simulink model "NeuromorphicDogGait_WalksBackwards"  (R2022b)
settings: Solver=ode4  StartTime=0.0  StopTime=10  FixedStep=1e-3  RelTol=1e-3
undefined symbols (not defined in the file): t1, t2, Vus0
libraries: vexv5lib x24, vexcommonlib x16, Vex_V5_Simulink_Expansion x8
(part 1 of 3)
settings Model: Creator=Serious Chimp  LastModifiedBy=Serious Chimp
settings DataIOCC: SaveFormat=StructureWithTime  InspectSignalLogs=on
settings OptimizationCC: EnhancedBackFolding=on  PassReuseOutputArgsAs=Individual arguments  ZeroExternalMemoryAtStartup=off  ZeroInternalMemoryAtStartup=off  MaxStackSize=64  OptimizeBlockOrder=speed  DifferentSizesBufferReuse=on  OptimizationCustomize=off  EfficientTunableParamExpr=on
settings DebuggingCC: ParameterTunabilityLossMsg=error
settings HardwareCC: ProdBitPerPointer=32  ProdBitPerSizeT=32  ProdBitPerPtrDiffT=32  ProdLargestAtomicInteger=Long  ProdLargestAtomicFloat=Double  ProdWordSize=32  ProdHWDeviceType=ARM Compatible->ARM Cortex  UseEmbeddedCoderFeatures=off
settings SFSimCC: MATLABDynamicMemAlloc=off
settings RTWCC: Description=Embedded Coder  SystemTargetFile=ert.tlc  HardwareBoard=VEX V5 Robot Brain  TLCOptions="-aInlineSetEventsForThisBaseRateFcn=TLC_FALSE -aSuppressMultiTaskScheduler=TLC_FALSE  -aRateBasedStepFcn=0"  TemplateMakefile=ert_default_tmf  Toolchain=GNU Tools for ARM Embedded Processors
settings CodeAppCC: ForceParamTrailComments=on  IgnoreCustomStorageClasses=off  OperatorAnnotations=on  SimulinkDataObjDesc=on  SFDataObjDesc=on  InsertBlockDesc=on
settings ERTTargetCC: SupportNonInlinedSFcns=on  ExtModeTransport=3  ExtModeStaticAlloc=on  ExtModeStaticAllocSize=2048  ExtModeMexFile=ext_xcp  ExtModeIntrfLevel=Level2 - Open

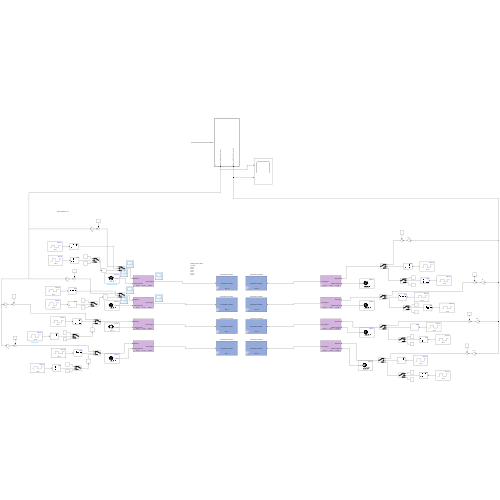
[thumbnail: Simulink's stored preview of the top-level diagram]
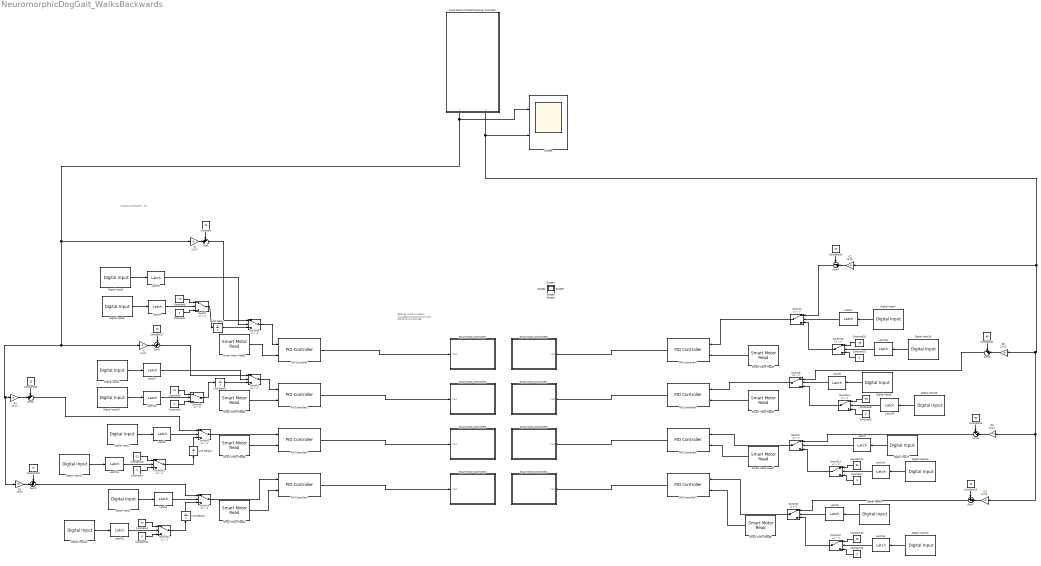
== system NeuromorphicDogGait_WalksBackwards ==
  note: Output amplitude ~ 19
  note: Settings used in videos:
      | k1=1200
      | k2=10
      | k3=10
      | C=15
      | D=23
      | t1=1.5
      | t2=190
  -C{,1..3} (4 alike) : Gain  Gain=15/19
  Constant : Constant  Value=70
  Constant{1..3,5,7,11..12,15} (8 alike) : Constant  Value=0
  Constant10 : Constant  Value=-13
  Constant13 : Constant  Value=15
  Constant14 : Constant  Value=90
  Constant16 : Constant  Value=-15
  Constant17 : Constant  Value=13
  Constant18 : Constant  Value=13
  Constant19 : Constant  Value=70
  Constant20 : Constant  Value=15
  Constant21 : Constant  Value=90
  Constant22 : Constant  Value=90
  Constant23 : Constant  Value=15
  Constant4 : Constant  Value=70
  Constant6 : Constant  Value=-90
  Constant8 : Constant  Value=-70
  Constant9 : Constant  Value=13
  D{,1..3} (4 alike) : Gain  Gain=23/19
  Digital Input{1..8} (8 alike) : vexv5lib/Sensors/Digital Input  smartPort3wire=None  port=H  SampleTime=0.2
  Digital Input{9..16} (8 alike) : vexv5lib/Sensors/Digital Input  smartPort3wire=None  port=A  SampleTime=0.2
  Latch{1..16} (16 alike) : vexcommonlib/Latch  output0=off  BlockPlatform=vexv5
      settings: LibrarySourceBlock=vexv5lib/Utilities/Latch
  PID Controller : Vex_V5_Simulink_Expansion/Core Blocks/PID Controller  KP=k1  KI=k3  KD=k2  LimitOutput=off  limitHigh=10  limitLow=10  AntiWindupMode=none  kb=0
      settings: SourceProductName=Vex V5 Simulink Expansion
  PID Controller{1..7} (7 alike) : Vex_V5_Simulink_Expansion/Core Blocks/PID Controller  KP=k1  KI=k3  KD=k2  LimitOutput=off  limitHigh=0  limitLow=0  AntiWindupMode=none  kb=0
      settings: SourceProductName=Vex V5 Simulink Expansion
  Quad-Centre (Closed Coupling) Oscillator : Subsystem  TreatAsAtomicUnit=on  mask{tau_s_A=t1, tau_us_A=t2, GB_A=-40, tau_s_B=t1, tau_us_B=t2, GB_B=-20, tau_s_C=t1, tau_us_C=t2, GB_C=-20, tau_s_D=t1, tau_us_D=t2, GB_D=-40, pain_threshold=2, pain_intensity=2, delay=0}
      mask prompts: tau_s_A "A - tau_s"; tau_us_A "A - tau_us"; GB_A "A - Inhibitory Synapse Threshold, GB_A"; tau_s_B "B - tau_s"; tau_us_B "B - tau_us"; GB_B "B - Inhibitory Synapse Threshold, GB_B"; tau_s_C "C - tau_s"; tau_us_C "C - tau_us"; GB_C "C - Inhibitory Synapse Threshold, GB_C"; tau_s_D "D - tau_s"; tau_us_D "D - tau_us"; GB_D "D - Inhibitory Synapse Threshold, GB_D"; pain_threshold "Range of Motion Pain Threshold, pain_threshold"; pain_intensity "Rang of Motion Intensity, pain_intensity"
  Scope6 : Scope  NumInputPorts=2
  Smart Motor Controller1 : Subsystem  AncestorBlock=Vex_V5_Simulink_Expansion/Core Blocks/Smart Motor Controller  mask(Smart Motor Controller){motorPort=19, OperationMode=Advanced Control, MotorBrakeMode=Coast}
      mask prompts: motorPort "Smart Port:"; OperationMode "Control Mode:"; MotorBrakeMode "Braking Mode:"
      mask help: Controls the Vex Smart Motor via the chosen method.
      mask TypeOptions motorPort: Advanced_SmartMotorWrite/motorPort
      mask TypeOptions OperationMode: Advanced_SmartMotorWrite/OperationMode
      mask TypeOptions MotorBrakeMode: Advanced_SmartMotorWrite/MotorBrakeMode
      mask DialogControl Container3 Prompt: Smart Motor Configuration
      mask Display:
      | %mode = get_param(gcb, 'control');
      | port = get_param(gcb, 'motorPort');
      | %text(0.3,0.45,[mode]);
      | 
      | text(0.5,0.5, 'Smart Motor Controller','HorizontalAlignment','center');
      | text(0.42,0.15, ['Port: ',port]);
  Smart Motor Controller2 : Subsystem  AncestorBlock=Vex_V5_Simulink_Expansion/Core Blocks/Smart Motor Controller  mask(Smart Motor Controller){motorPort=9, OperationMode=Advanced Control, MotorBrakeMode=Coast}
      mask prompts: motorPort "Smart Port:"; OperationMode "Control Mode:"; MotorBrakeMode "Braking Mode:"
      mask help: Controls the Vex Smart Motor via the chosen method.
      mask TypeOptions motorPort: Advanced_SmartMotorWrite/motorPort
      mask TypeOptions OperationMode: Advanced_SmartMotorWrite/OperationMode
      mask TypeOptions MotorBrakeMode: Advanced_SmartMotorWrite/MotorBrakeMode
      mask DialogControl Container3 Prompt: Smart Motor Configuration
      mask Display:
      | %mode = get_param(gcb, 'control');
      | port = get_param(gcb, 'motorPort');
      | %text(0.3,0.45,[mode]);
      | 
      | text(0.5,0.5, 'Smart Motor Controller','HorizontalAlignment','center');
      | text(0.42,0.15, ['Port: ',port]);
  Smart Motor Controller3 : Subsystem  AncestorBlock=Vex_V5_Simulink_Expansion/Core Blocks/Smart Motor Controller  mask(Smart Motor Controller){motorPort=1, OperationMode=Advanced Control, MotorBrakeMode=Coast}
      mask prompts: motorPort "Smart Port:"; OperationMode "Control Mode:"; MotorBrakeMode "Braking Mode:"
      mask help: Controls the Vex Smart Motor via the chosen method.
      mask TypeOptions motorPort: Advanced_SmartMotorWrite/motorPort
      mask TypeOptions OperationMode: Advanced_SmartMotorWrite/OperationMode
      mask TypeOptions MotorBrakeMode: Advanced_SmartMotorWrite/MotorBrakeMode
      mask DialogControl Container3 Prompt: Smart Motor Configuration
      mask Display:
      | %mode = get_param(gcb, 'control');
      | port = get_param(gcb, 'motorPort');
      | %text(0.3,0.45,[mode]);
      | 
      | text(0.5,0.5, 'Smart Motor Controller','HorizontalAlignment','center');
      | text(0.42,0.15, ['Port: ',port]);
  Smart Motor Controller4 : Subsystem  AncestorBlock=Vex_V5_Simulink_Expansion/Core Blocks/Smart Motor Controller  mask(Smart Motor Controller){motorPort=11, OperationMode=Advanced Control, MotorBrakeMode=Coast}
      mask prompts: motorPort "Smart Port:"; OperationMode "Control Mode:"; MotorBrakeMode "Braking Mode:"
      mask help: Controls the Vex Smart Motor via the chosen method.
      mask TypeOptions motorPort: Advanced_SmartMotorWrite/motorPort
      mask TypeOptions OperationMode: Advanced_SmartMotorWrite/OperationMode
      mask TypeOptions MotorBrakeMode: Advanced_SmartMotorWrite/MotorBrakeMode
      mask DialogControl Container3 Prompt: Smart Motor Configuration
      mask Display:
      | %mode = get_param(gcb, 'control');
      | port = get_param(gcb, 'motorPort');
      | %text(0.3,0.45,[mode]);
      | 
      | text(0.5,0.5, 'Smart Motor Controller','HorizontalAlignment','center');
      | text(0.42,0.15, ['Port: ',port]);
  Smart Motor Controller5 : Subsystem  AncestorBlock=Vex_V5_Simulink_Expansion/Core Blocks/Smart Motor Controller  mask(Smart Motor Controller){motorPort=2, OperationMode=Advanced Control, MotorBrakeMode=Coast}
      mask prompts: motorPort "Smart Port:"; OperationMode "Control Mode:"; MotorBrakeMode "Braking Mode:"
      mask help: Controls the Vex Smart Motor via the chosen method.
      mask TypeOptions motorPort: Advanced_SmartMotorWrite/motorPort
      mask TypeOptions OperationMode: Advanced_SmartMotorWrite/OperationMode
      mask TypeOptions MotorBrakeMode: Advanced_SmartMotorWrite/MotorBrakeMode
      mask DialogControl Container3 Prompt: Smart Motor Configuration
      mask Display:
      | %mode = get_param(gcb, 'control');
      | port = get_param(gcb, 'motorPort');
      | %text(0.3,0.45,[mode]);
      | 
      | text(0.5,0.5, 'Smart Motor Controller','HorizontalAlignment','center');
      | text(0.42,0.15, ['Port: ',port]);
  Smart Motor Controller6 : Subsystem  AncestorBlock=Vex_V5_Simulink_Expansion/Core Blocks/Smart Motor Controller  mask(Smart Motor Controller){motorPort=12, OperationMode=Advanced Control, MotorBrakeMode=Coast}
      mask prompts: motorPort "Smart Port:"; OperationMode "Control Mode:"; MotorBrakeMode "Braking Mode:"
      mask help: Controls the Vex Smart Motor via the chosen method.
      mask TypeOptions motorPort: Advanced_SmartMotorWrite/motorPort
      mask TypeOptions OperationMode: Advanced_SmartMotorWrite/OperationMode
      mask TypeOptions MotorBrakeMode: Advanced_SmartMotorWrite/MotorBrakeMode
      mask DialogControl Container3 Prompt: Smart Motor Configuration
      mask Display:
      | %mode = get_param(gcb, 'control');
      | port = get_param(gcb, 'motorPort');
      | %text(0.3,0.45,[mode]);
      | 
      | text(0.5,0.5, 'Smart Motor Controller','HorizontalAlignment','center');
      | text(0.42,0.15, ['Port: ',port]);
  Smart Motor Controller7 : Subsystem  AncestorBlock=Vex_V5_Simulink_Expansion/Core Blocks/Smart Motor Controller  mask(Smart Motor Controller){motorPort=10, OperationMode=Advanced Control, MotorBrakeMode=Coast}
      mask prompts: motorPort "Smart Port:"; OperationMode "Control Mode:"; MotorBrakeMode "Braking Mode:"
      mask help: Controls the Vex Smart Motor via the chosen method.
      mask TypeOptions motorPort: Advanced_SmartMotorWrite/motorPort
      mask TypeOptions OperationMode: Advanced_SmartMotorWrite/OperationMode
      mask TypeOptions MotorBrakeMode: Advanced_SmartMotorWrite/MotorBrakeMode
      mask DialogControl Container3 Prompt: Smart Motor Configuration
      mask Display:
      | %mode = get_param(gcb, 'control');
      | port = get_param(gcb, 'motorPort');
      | %text(0.3,0.45,[mode]);
      | 
      | text(0.5,0.5, 'Smart Motor Controller','HorizontalAlignment','center');
      | text(0.42,0.15, ['Port: ',port]);
  Smart Motor Controller8 : Subsystem  AncestorBlock=Vex_V5_Simulink_Expansion/Core Blocks/Smart Motor Controller  mask(Smart Motor Controller){motorPort=20, OperationMode=Advanced Control, MotorBrakeMode=Coast}
      mask prompts: motorPort "Smart Port:"; OperationMode "Control Mode:"; MotorBrakeMode "Braking Mode:"
      mask help: Controls the Vex Smart Motor via the chosen method.
      mask TypeOptions motorPort: Advanced_SmartMotorWrite/motorPort
      mask TypeOptions OperationMode: Advanced_SmartMotorWrite/OperationMode
      mask TypeOptions MotorBrakeMode: Advanced_SmartMotorWrite/MotorBrakeMode
      mask DialogControl Container3 Prompt: Smart Motor Configuration
      mask Display:
      | %mode = get_param(gcb, 'control');
      | port = get_param(gcb, 'motorPort');
      | %text(0.3,0.45,[mode]);
      | 
      | text(0.5,0.5, 'Smart Motor Controller','HorizontalAlignment','center');
      | text(0.42,0.15, ['Port: ',port]);
  Smart Motor Read1 : vexv5lib/Sensors/Smart Motor Read  motorPort=10  EncoderUnit=Degrees  resetOption=No reset  additionalOutput=off  SampleTime=0.01
  Smart Motor Read2 : vexv5lib/Sensors/Smart Motor Read  motorPort=9  EncoderUnit=Degrees  resetOption=No reset  additionalOutput=off  SampleTime=0.01
  Smart Motor Read3 : vexv5lib/Sensors/Smart Motor Read  motorPort=2  EncoderUnit=Degrees  resetOption=No reset  additionalOutput=off  SampleTime=0.01
  Smart Motor Read4 : vexv5lib/Sensors/Smart Motor Read  motorPort=1  EncoderUnit=Degrees  resetOption=No reset  additionalOutput=off  SampleTime=0.01
  Smart Motor Read5 : vexv5lib/Sensors/Smart Motor Read  motorPort=20  EncoderUnit=Degrees  resetOption=No reset  additionalOutput=off  SampleTime=0.01
  Smart Motor Read6 : vexv5lib/Sensors/Smart Motor Read  motorPort=19  EncoderUnit=Degrees  resetOption=No reset  additionalOutput=off  SampleTime=0.01
  Smart Motor Read7 : vexv5lib/Sensors/Smart Motor Read  motorPort=12  EncoderUnit=Degrees  resetOption=No reset  additionalOutput=off  SampleTime=0.01
  Smart Motor Read8 : vexv5lib/Sensors/Smart Motor Read  motorPort=11  EncoderUnit=Degrees  resetOption=No reset  additionalOutput=off  SampleTime=0.01
  Sum{,2,4..5} (4 alike) : Sum  Inputs=-+|
  Sum{1,3,6..7} (4 alike) : Sum  Inputs=++|
  Switch{,1..15} (16 alike) : Switch  Criteria=u2 > Threshold  SaturateOnIntegerOverflow=off  InputSameDT=off
  Unit Delay{,1..3} (4 alike) : UnitDelay  SampleTime=-1  HasFrameUpgradeWarning=on
  Scope{,1..5} (6 alike) : Scope
  wires:
  Smart Motor Read1/1 -> PID Controller/2
  Smart Motor Read2/1 -> PID Controller1/2
  Smart Motor Read4/1 -> PID Controller3/2
  Smart Motor Read3/1 -> PID Controller2/2
  Smart Motor Read5/1 -> PID Controller4/2
  Smart Motor Read6/1 -> PID Controller5/2
  Smart Motor Read7/1 -> PID Controller6/2
  Smart Motor Read8/1 -> PID Controller7/2
  Digital Input5/1 -> Latch5/1
  Latch5/1 -> Switch5/2
  Switch5/1 -> PID Controller/1
  Switch9/1 -> Unit Delay1/1
  Digital Input1/1 -> Latch1/1
  Latch1/1 -> Switch1/2
  Switch1/1 -> PID Controller1/1
  Digital Input2/1 -> Latch2/1
  Latch2/1 -> Switch2/2
  Switch2/1 -> PID Controller2/1
  Digital Input3/1 -> Latch3/1
  Latch3/1 -> Switch3/2
  Switch3/1 -> PID Controller3/1
  Digital Input4/1 -> Latch4/1
  Latch4/1 -> Switch4/2
  Switch4/1 -> PID Controller4/1
  Digital Input6/1 -> Latch6/1
  Latch6/1 -> Switch6/2
  Switch6/1 -> PID Controller5/1
  Digital Input7/1 -> Latch7/1
  Latch7/1 -> Switch7/2
  Switch7/1 -> PID Controller6/1
  Digital Input8/1 -> Latch8/1
  Latch8/1 -> Switch8/2
  Switch8/1 -> PID Controller7/1
  Constant1/1 -> Switch/3
  Constant8/1 -> Switch/1
  Digital Input9/1 -> Latch9/1
  Latch9/1 -> Switch/2
  Constant9/1 -> Switch9/1
  Latch10/1 -> Switch9/2
  Constant2/1 -> Switch9/3
  Digital Input10/1 -> Latch10/1
  Constant10/1 -> Switch10/1
  Latch11/1 -> Switch10/2
  Constant3/1 -> Switch10/3
  Digital Input11/1 -> Latch11/1
  Constant11/1 -> Switch11/3
  Constant4/1 -> Switch11/1
  Digital Input12/1 -> Latch12/1
  Latch12/1 -> Switch11/2
  Digital Input13/1 -> Latch13/1
  Constant13/1 -> Switch12/1
  Constant12/1 -> Switch12/3
  Latch13/1 -> Switch12/2
  Digital Input14/1 -> Latch14/1
  Constant14/1 -> Switch13/1
  Constant7/1 -> Switch13/3
  Latch14/1 -> Switch13/2
  Digital Input15/1 -> Latch15/1
  Constant6/1 -> Switch14/1
  Constant5/1 -> Switch14/3
  Latch15/1 -> Switch14/2
  Digital Input16/1 -> Latch16/1
  Constant16/1 -> Switch15/1
  Constant15/1 -> Switch15/3
  Latch16/1 -> Switch15/2
  Switch/1 -> Unit Delay/1
  Switch10/1 -> Unit Delay2/1
  Unit Delay2/1 -> Switch2/3
  Unit Delay1/1 -> Switch1/3
  Unit Delay/1 -> Switch5/3
  Switch13/1 -> Switch7/3
  Switch14/1 -> Switch6/3
  Unit Delay3/1 -> Switch3/3
  Switch11/1 -> Unit Delay3/1
  Switch15/1 -> Switch4/3
  Switch12/1 -> Switch8/3
  PID Controller/1 -> Smart Motor Controller7/1(" Input")
  PID Controller1/1 -> Smart Motor Controller2/1(" Input")
  PID Controller2/1 -> Smart Motor Controller5/1(" Input")
  PID Controller3/1 -> Smart Motor Controller3/1(" Input")
  PID Controller4/1 -> Smart Motor Controller8/1(" Input")
  PID Controller5/1 -> Smart Motor Controller1/1(" Input")
  PID Controller6/1 -> Smart Motor Controller6/1(" Input")
  PID Controller7/1 -> Smart Motor Controller4/1(" Input")
  Constant/1 -> Sum/1
  D/1 -> Sum/2
  Sum/1 -> Switch5/1
  Constant17/1 -> Sum1/1
  -C/1 -> Sum1/2
  Sum1/1 -> Switch1/1
  Constant18/1 -> Sum2/1
  -C1/1 -> Sum2/2
  Sum2/1 -> Switch2/1
  Constant19/1 -> Sum3/1
  D1/1 -> Sum3/2
  Sum3/1 -> Switch3/1
  Constant20/1 -> Sum4/1
  -C2/1 -> Sum4/2
  Constant21/1 -> Sum5/1
  D2/1 -> Sum5/2
  Sum5/1 -> Switch6/1
  D3/1 -> Sum6/2
  Constant22/1 -> Sum6/1
  Sum6/1 -> Switch7/1
  Constant23/1 -> Sum7/1
  -C3/1 -> Sum7/2
  Sum7/1 -> Switch8/1
  Sum4/1 -> Switch4/1
  Quad-Centre (Closed Coupling) Oscillator/1(Neuromorphic Waveform Phase 0) -> Scope6/1, D1/1, -C1/1, -C/1, D/1
  Quad-Centre (Closed Coupling) Oscillator/2(Neuromorphic Waveform Phase 180) -> -C2/1, -C3/1, D3/1, D2/1, Scope6/2

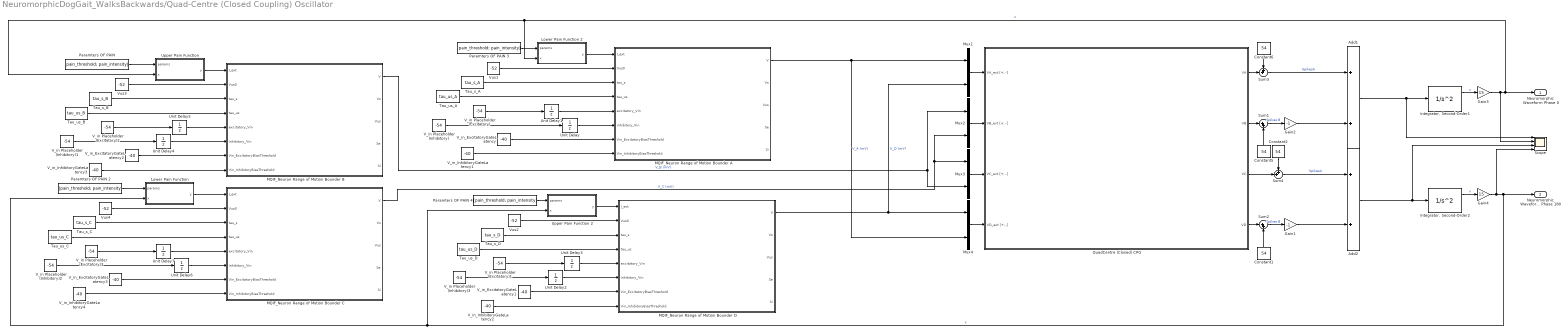
== system NeuromorphicDogGait_WalksBackwards/Quad-Centre (Closed Coupling) Oscillator ==
  Add1 : Sum
  Add2 : Sum
  Constant{1..2,5..6} (4 alike) : Constant  Value=54
  Gain1 : Gain  Gain=-1
  Gain2 : Gain  Gain=-1
  Gain3 : Gain  Gain=15
  Gain4 : Gain  Gain=15
  "Integrator, Second-Order1" : SecondOrderIntegrator
  "Integrator, Second-Order2" : SecondOrderIntegrator
  Lower Pain Function : MATLAB Function  TreatAsAtomicUnit=on
  Lower Pain Function 2 : MATLAB Function  TreatAsAtomicUnit=on
  MQIF_Neuron Range of Motion Bounder A : Subsystem  TreatAsAtomicUnit=on  mask{V0=-52, Vs0=-50, V_threshold=20, V_reset=-45, Vs_reset=7.5, delta_Vus=1.7, g_f=1.0, g_s=0.5, g_us=0.015, C=0.82, Ve_syn=0, Vi_syn=-80, g_syn_excitatory=45, g_syn_inhibitory=45, tauSyn_excitatory=7, tauSyn_inhibitory=7, k=250}
      mask prompts: V0 "Equilibrium V0"; Vs0 "Equilibrium Vs0"; V_threshold "Threshold for Spike, V_thresh"; V_reset "After-spike Reset Votlage, V_r"; Vs_reset "After-spike Reset Vs, Vs_r"; delta_Vus "Vus After-spike Memory, delta_Vus"; g_f "I Conductance, g_f"; g_s "I_us Conductance, g_s"; g_us "I_us Conductance, g_us"; C "Capacitance, C"; Ve_syn "Equilibrium Inhibitory Synapse Voltage, Ve_syn"; Vi_syn "Equilibrium Inhibitory Synapse Voltage, Vi_syn"; g_syn_excitatory "Excitatory Synapse Conductance, g_syn_excitatory"; g_syn_inhibitory "Inhibitory Synapse Conductance, g_syn_inhibitory"; tauSyn_excitatory "Excitatory Synapse Time Constant, tauSyn_excitatory"; tauSyn_inhibitory "Inhibitory Synapse Time Constant, tauSyn_inhibitory"; k "Speed/Rate Constant, k"
      mask DialogControl NeuronStateVariables Prompt: Parameters
  MQIF_Neuron Range of Motion Bounder B : Subsystem  TreatAsAtomicUnit=on  mask{V0=-52, Vs0=-50, V_threshold=20, V_reset=-45, Vs_reset=7.5, delta_Vus=1.7, g_f=1.0, g_s=0.5, g_us=0.015, C=0.82, Ve_syn=0, Vi_syn=-80, g_syn_excitatory=45, g_syn_inhibitory=45, tauSyn_excitatory=7, tauSyn_inhibitory=7, k=250}
      mask prompts: V0 "Equilibrium V0"; Vs0 "Equilibrium Vs0"; V_threshold "Threshold for Spike, V_thresh"; V_reset "After-spike Reset Votlage, V_r"; Vs_reset "After-spike Reset Vs, Vs_r"; delta_Vus "Vus After-spike Memory, delta_Vus"; g_f "I Conductance, g_f"; g_s "I_us Conductance, g_s"; g_us "I_us Conductance, g_us"; C "Capacitance, C"; Ve_syn "Equilibrium Inhibitory Synapse Voltage, Ve_syn"; Vi_syn "Equilibrium Inhibitory Synapse Voltage, Vi_syn"; g_syn_excitatory "Excitatory Synapse Conductance, g_syn_excitatory"; g_syn_inhibitory "Inhibitory Synapse Conductance, g_syn_inhibitory"; tauSyn_excitatory "Excitatory Synapse Time Constant, tauSyn_excitatory"; tauSyn_inhibitory "Inhibitory Synapse Time Constant, tauSyn_inhibitory"; k "Speed/Rate Constant, k"
      mask DialogControl NeuronStateVariables Prompt: Parameters
  MQIF_Neuron Range of Motion Bounder C : Subsystem  TreatAsAtomicUnit=on  mask{V0=-52, Vs0=-50, V_threshold=20, V_reset=-45, Vs_reset=7.5, delta_Vus=1.7, g_f=1.0, g_s=0.5, g_us=0.015, C=0.82, Ve_syn=0, Vi_syn=-80, g_syn_excitatory=45, g_syn_inhibitory=45, tauSyn_excitatory=7, tauSyn_inhibitory=7, k=250}
      mask prompts: V0 "Equilibrium V0"; Vs0 "Equilibrium Vs0"; V_threshold "Threshold for Spike, V_thresh"; V_reset "After-spike Reset Votlage, V_r"; Vs_reset "After-spike Reset Vs, Vs_r"; delta_Vus "Vus After-spike Memory, delta_Vus"; g_f "I Conductance, g_f"; g_s "I_us Conductance, g_s"; g_us "I_us Conductance, g_us"; C "Capacitance, C"; Ve_syn "Equilibrium Inhibitory Synapse Voltage, Ve_syn"; Vi_syn "Equilibrium Inhibitory Synapse Voltage, Vi_syn"; g_syn_excitatory "Excitatory Synapse Conductance, g_syn_excitatory"; g_syn_inhibitory "Inhibitory Synapse Conductance, g_syn_inhibitory"; tauSyn_excitatory "Excitatory Synapse Time Constant, tauSyn_excitatory"; tauSyn_inhibitory "Inhibitory Synapse Time Constant, tauSyn_inhibitory"; k "Speed/Rate Constant, k"
      mask DialogControl NeuronStateVariables Prompt: Parameters
  MQIF_Neuron Range of Motion Bounder D : Subsystem  TreatAsAtomicUnit=on  mask{V0=-52, Vs0=-50, V_threshold=20, V_reset=-45, Vs_reset=7.5, delta_Vus=1.7, g_f=1.0, g_s=0.5, g_us=0.015, C=0.82, Ve_syn=0, Vi_syn=-80, g_syn_excitatory=45, g_syn_inhibitory=45, tauSyn_excitatory=7, tauSyn_inhibitory=7, k=250}
      mask prompts: V0 "Equilibrium V0"; Vs0 "Equilibrium Vs0"; V_threshold "Threshold for Spike, V_thresh"; V_reset "After-spike Reset Votlage, V_r"; Vs_reset "After-spike Reset Vs, Vs_r"; delta_Vus "Vus After-spike Memory, delta_Vus"; g_f "I Conductance, g_f"; g_s "I_us Conductance, g_s"; g_us "I_us Conductance, g_us"; C "Capacitance, C"; Ve_syn "Equilibrium Inhibitory Synapse Voltage, Ve_syn"; Vi_syn "Equilibrium Inhibitory Synapse Voltage, Vi_syn"; g_syn_excitatory "Excitatory Synapse Conductance, g_syn_excitatory"; g_syn_inhibitory "Inhibitory Synapse Conductance, g_syn_inhibitory"; tauSyn_excitatory "Excitatory Synapse Time Constant, tauSyn_excitatory"; tauSyn_inhibitory "Inhibitory Synapse Time Constant, tauSyn_inhibitory"; k "Speed/Rate Constant, k"
      mask DialogControl NeuronStateVariables Prompt: Parameters
  Mux{1..4} (4 alike) : Mux  Inputs=2
  Paramters OF PAIN : Constant  Value=[pain_threshold; pain_intensity]
  Paramters OF PAIN 2 : Constant  Value=[pain_threshold; pain_intensity]
  Paramters OF PAIN 3 : Constant  Value=[pain_threshold; pain_intensity]
  Paramters OF PAIN 4 : Constant  Value=[pain_threshold; pain_intensity]
  QuadCentre (Closed) CPG : Subsystem  TreatAsAtomicUnit=on  mask{tau_s_A=t1, tau_us_A=t2, gSyn_excitatory_A=0.5, gSyn_inhibitory_A=0.5, tauSyn_excitatory_A=50, tauSyn_inhibitory_A=50, GB_A=-40, tau_s_B=t1, tau_us_B=t2, gSyn_excitatory_B=0.5, gSyn_inhibitory_B=0.5, tauSyn_excitatory_B=50, tauSyn_inhibitory_B=50, GB_B=-35, tau_s_C=t1, tau_us_C=t2, gSyn_excitatory_C=0.5, gSyn_inhibitory_C=0.5, tauSyn_excitatory_C=50, tauSyn_inhibitory_C=50, GB_C=-35, tau_s_D=t1, tau_us_D=t2, gSyn_excitatory_D=0.5, gSyn_inhibitory_D=0.5, tauSyn_excitatory_D=50, tauSyn_inhibitory_D=50, GB_D=-40, GB_excitatory=-40, R=200}
      mask prompts: tau_s_A "A - tau_s"; tau_us_A "A - tau_us"; gSyn_excitatory_A "A - Excitatory Synaptic Conductance, gSyn_excitatory"; gSyn_inhibitory_A "A - Inhibitory Synaptic Conductance, gSyn_inhibitory"; tauSyn_excitatory_A "A - Excitatory Synaptic Time Constant, tauSyn_excitatory"; tauSyn_inhibitory_A "A - Inhibitory Synaptic Time Constant, tauSyn_inhibitory"; GB_A "A - Inhibitory Synapse Threshold, GB_A"; tau_s_B "B - tau_s"; tau_us_B "B - tau_us"; gSyn_excitatory_B "B - Excitatory Synaptic Conductance, gSyn_excitatory"; gSyn_inhibitory_B "B - Inhibitory Synaptic Conductance, gSyn_inhibitory"; tauSyn_excitatory_B "B - Excitatory Synaptic Time Constant, tauSyn_excitatory"; tauSyn_inhibitory_B "B - Inhibitory Synaptic Time Constant, tauSyn_inhibitory"; GB_B "B - Inhibitory Synapse Threshold, GB_B"; tau_s_C "C - tau_s"; tau_us_C "C - tau_us"; gSyn_excitatory_C "C - Excitatory Synaptic Conductance, gSyn_excitatory"; gSyn_inhibitory_C "C - Inhibitory Synaptic Conductance, gSyn_inhibitory"; tauSyn_excitatory_C "C - Excitatory Synaptic Time Constant, tauSyn_excitatory"; tauSyn_inhibitory_C "C - Inhibitory Synaptic Time Constant, tauSyn_inhibitory"; GB_C "C - Inhibitory Synapse Threshold, GB_C"; tau_s_D "D - tau_s"; tau_us_D "D - tau_us"; gSyn_excitatory_D "D - Excitatory Synaptic Conductance, gSyn_excitatory"; gSyn_inhibitory_D "D - Inhibitory Synaptic Conductance, gSyn_inhibitory"; tauSyn_excitatory_D "D - Excitatory Synaptic Time Constant, tauSyn_excitatory"; tauSyn_inhibitory_D "D - Inhibitory Synaptic Time Constant, tauSyn_inhibitory"; GB_D "D - Inhibitory Synapse Threshold, GB_D"; GB_excitatory "Excitatory Synapse Gate Threshold, GB_excitatory"; R "Coupling Resistance, R"
      mask Display: image('$imagefile'); % Use "Edit Image" on toolstrip to change.
  Scope : Scope  NumInputPorts=4
  Sum1 : Sum  Inputs=|++
  Sum2 : Sum  Inputs=|++
  Sum3 : Sum  Inputs=++|
  Sum4 : Sum  Inputs=++|
  Tau_s_A : Constant  Value=tau_s_A
  Tau_s_B : Constant  Value=tau_s_B
  Tau_s_C : Constant  Value=tau_s_C
  Tau_s_D : Constant  Value=tau_s_D
  Tau_us_A : Constant  Value=tau_us_A
  Tau_us_B : Constant  Value=tau_us_B
  Tau_us_C : Constant  Value=tau_us_C
  Tau_us_D : Constant  Value=tau_us_D
  Unit Delay{,1..7} (8 alike) : UnitDelay  InitialCondition=-54  SampleTime=-1  HasFrameUpgradeWarning=on
  Upper Pain Function : MATLAB Function  TreatAsAtomicUnit=on
  Upper Pain Function 2 : MATLAB Function  TreatAsAtomicUnit=on
  V_in Placeholder (Excitatory){,1..3} (4 alike) : Constant  Value=-54
  V_in Placeholder (Inhibitory){,1..3} (4 alike) : Constant  Value=-54
  V_in_ExcitatoryGateLatency{,1..3} (4 alike) : Constant  Value=-40
  V_in_InhibitoryGateLatency{1..4} (4 alike) : Constant  Value=-40
  Vus{1..4} (4 alike) : Constant  Value=-52
  Neuromorphic Waveform Phase 0 : Outport
  Neuromorphic Waveform Phase 180 : Outport  Port=2
  wires:
  Constant5/1 -> Sum1/2
  MQIF_Neuron Range of Motion Bounder D/1(V) -> Mux1/2, Mux4/1  "V_D (mV)"
  V_in_ExcitatoryGateLatency/1 -> MQIF_Neuron Range of Motion Bounder A/7(Vin_ExcitatoryBiasThreshold)
  V_in Placeholder (Inhibitory)3/1 -> Unit Delay2/1
  Gain2/1 -> Add1/2
  V_in_InhibitoryGateLatency2/1 -> MQIF_Neuron Range of Motion Bounder D/8(Vin_InhibitoryBiasThreshold)
  Vus1/1 -> MQIF_Neuron Range of Motion Bounder A/2(Vus0)
  V_in Placeholder (Excitatory)/1 -> Unit Delay1/1
  Unit Delay2/1 -> MQIF_Neuron Range of Motion Bounder D/6(inhibitory_Vin)
  Unit Delay/1 -> MQIF_Neuron Range of Motion Bounder A/6(inhibitory_Vin)
  Tau_s_D/1 -> MQIF_Neuron Range of Motion Bounder D/3(tau_s)
  Vus2/1 -> MQIF_Neuron Range of Motion Bounder D/2(Vus0)
  V_in Placeholder (Inhibitory)/1 -> Unit Delay/1
  "Integrator, Second-Order1"/1 -> Gain3/1  "x"
  V_in_ExcitatoryGateLatency1/1 -> MQIF_Neuron Range of Motion Bounder D/7(Vin_ExcitatoryBiasThreshold)
  Sum3/1 -> Add1/1  "SpikesA"
  QuadCentre (Closed) CPG/1(VA) -> Sum3/2
  V_in Placeholder (Excitatory)1/1 -> Unit Delay3/1
  Tau_us_A/1 -> MQIF_Neuron Range of Motion Bounder A/4(tau_us)
  V_in_InhibitoryGateLatency1/1 -> MQIF_Neuron Range of Motion Bounder A/8(Vin_InhibitoryBiasThreshold)
  Unit Delay1/1 -> MQIF_Neuron Range of Motion Bounder A/5(excitatory_Vin)
  MQIF_Neuron Range of Motion Bounder A/1(V) -> Mux4/2, Mux1/1  "V_A (mV)"
  Tau_s_A/1 -> MQIF_Neuron Range of Motion Bounder A/3(tau_s)
  Lower Pain Function 2/1(y) -> MQIF_Neuron Range of Motion Bounder A/1(I_ext)
  Tau_us_D/1 -> MQIF_Neuron Range of Motion Bounder D/4(tau_us)
  QuadCentre (Closed) CPG/2(VB) -> Sum1/1
  Sum1/1 -> Gain2/1  "Spikes B"
  Unit Delay3/1 -> MQIF_Neuron Range of Motion Bounder D/5(excitatory_Vin)
  Constant6/1 -> Sum3/1
  Upper Pain Function 2/1(y) -> MQIF_Neuron Range of Motion Bounder D/1(I_ext)
  QuadCentre (Closed) CPG/3(VC) -> Sum4/2
  Gain1/1 -> Add2/2
  Sum2/1 -> Gain1/1  "Spikes B"
  QuadCentre (Closed) CPG/4(VD) -> Sum2/1
  Constant2/1 -> Sum4/1
  "Integrator, Second-Order2"/1 -> Gain4/1  "x"
  Constant1/1 -> Sum2/2
  Sum4/1 -> Add2/1  "SpikesA"
  Mux1/1 -> QuadCentre (Closed) CPG/1(VA_ext [+; -])
  Mux4/1 -> QuadCentre (Closed) CPG/4(VD_ext [+; -])
  Upper Pain Function/1(y) -> MQIF_Neuron Range of Motion Bounder B/1(I_ext)
  Unit Delay4/1 -> MQIF_Neuron Range of Motion Bounder B/6(inhibitory_Vin)
  V_in Placeholder (Excitatory)2/1 -> Unit Delay5/1
  Tau_us_B/1 -> MQIF_Neuron Range of Motion Bounder B/4(tau_us)
  Gain3/1 -> Scope/2, Neuromorphic Waveform Phase 0/1, Lower Pain Function 2/2(x), Upper Pain Function/2(x)  "x"
  Vus3/1 -> MQIF_Neuron Range of Motion Bounder B/2(Vus0)
  V_in_ExcitatoryGateLatency2/1 -> MQIF_Neuron Range of Motion Bounder B/7(Vin_ExcitatoryBiasThreshold)
  V_in Placeholder (Inhibitory)1/1 -> Unit Delay4/1
  Unit Delay5/1 -> MQIF_Neuron Range of Motion Bounder B/5(excitatory_Vin)
  Tau_s_B/1 -> MQIF_Neuron Range of Motion Bounder B/3(tau_s)
  V_in_InhibitoryGateLatency3/1 -> MQIF_Neuron Range of Motion Bounder B/8(Vin_InhibitoryBiasThreshold)
  Mux2/1 -> QuadCentre (Closed) CPG/2(VB_ext [+; -])
  MQIF_Neuron Range of Motion Bounder B/1(V) -> Mux2/1, Mux3/2  "V_B (mV)"
  Lower Pain Function/1(y) -> MQIF_Neuron Range of Motion Bounder C/1(I_ext)
  Gain4/1 -> Neuromorphic Waveform Phase 180/1, Upper Pain Function 2/2(x), Lower Pain Function/2(x), Scope/4  "x"
  Unit Delay7/1 -> MQIF_Neuron Range of Motion Bounder C/5(excitatory_Vin)
  V_in Placeholder (Inhibitory)2/1 -> Unit Delay6/1
  V_in_InhibitoryGateLatency4/1 -> MQIF_Neuron Range of Motion Bounder C/8(Vin_InhibitoryBiasThreshold)
  Tau_s_C/1 -> MQIF_Neuron Range of Motion Bounder C/3(tau_s)
  V_in Placeholder (Excitatory)3/1 -> Unit Delay7/1
  Vus4/1 -> MQIF_Neuron Range of Motion Bounder C/2(Vus0)
  V_in_ExcitatoryGateLatency3/1 -> MQIF_Neuron Range of Motion Bounder C/7(Vin_ExcitatoryBiasThreshold)
  Unit Delay6/1 -> MQIF_Neuron Range of Motion Bounder C/6(inhibitory_Vin)
  Tau_us_C/1 -> MQIF_Neuron Range of Motion Bounder C/4(tau_us)
  MQIF_Neuron Range of Motion Bounder C/1(V) -> Mux2/2, Mux3/1  "V_C (mV)"
  Mux3/1 -> QuadCentre (Closed) CPG/3(VC_ext [+; -])
  Add2/1 -> Scope/3, "Integrator, Second-Order2"/1
  Add1/1 -> Scope/1, "Integrator, Second-Order1"/1
  Paramters OF PAIN/1 -> Upper Pain Function/1(params)
  Paramters OF PAIN 3/1 -> Lower Pain Function 2/1(params)
  Paramters OF PAIN 2/1 -> Lower Pain Function/1(params)
  Paramters OF PAIN 4/1 -> Upper Pain Function 2/1(params)

== system NeuromorphicDogGait_WalksBackwards/Smart Motor Controller1 ==
  " Input" : Inport
  Advanced_SmartMotorWrite : MATLABSystem  System=Advanced_SmartMotorWrite  motorPort=19  scaleFactor=36:1  MotorBrakeMode=Coast  OperationMode=Advanced Control
      mask Type: Advanced_SmartMotorWrite
      mask Display:
      | color('white');
      | plot([100,100,100,100]*1,[100,100,100,100]*1);
      | plot([100,100,100,100]*0,[100,100,100,100]*0);
      | color('black');
      | image(fullfile(codertarget.vexv5.internal.getSpPkgRootDir, 'resources', 'vex-v5-motor2.png'),'center');
      | patch([0.8, 0.8, 1, 1], [0.82857, 1, 1, 0.82857], [1, 1, 1]);
      | color('blue');
      | text(99, 92, 'VEX V5 ', 'horizontalAlignment', 'right');
      | color('black');
      | text(62,12,'Port: 19','horizontalAlignment','center');
      | 
      | port_label('Input',1,'Voltage(mV)');
  wires:
  " Input"/1 -> Advanced_SmartMotorWrite/1

== system NeuromorphicDogGait_WalksBackwards/Smart Motor Controller2 ==
  " Input" : Inport
  Advanced_SmartMotorWrite : MATLABSystem  System=Advanced_SmartMotorWrite  motorPort=9  scaleFactor=36:1  MotorBrakeMode=Coast  OperationMode=Advanced Control
      mask Type: Advanced_SmartMotorWrite
      mask Display:
      | color('white');
      | plot([100,100,100,100]*1,[100,100,100,100]*1);
      | plot([100,100,100,100]*0,[100,100,100,100]*0);
      | color('black');
      | image(fullfile(codertarget.vexv5.internal.getSpPkgRootDir, 'resources', 'vex-v5-motor2.png'),'center');
      | patch([0.8, 0.8, 1, 1], [0.82857, 1, 1, 0.82857], [1, 1, 1]);
      | color('blue');
      | text(99, 92, 'VEX V5 ', 'horizontalAlignment', 'right');
      | color('black');
      | text(62,12,'Port: 9','horizontalAlignment','center');
      | 
      | port_label('Input',1,'Voltage(mV)');
  wires:
  " Input"/1 -> Advanced_SmartMotorWrite/1

== system NeuromorphicDogGait_WalksBackwards/Smart Motor Controller3 ==
  " Input" : Inport
  Advanced_SmartMotorWrite : MATLABSystem  System=Advanced_SmartMotorWrite  motorPort=1  scaleFactor=36:1  MotorBrakeMode=Coast  OperationMode=Advanced Control
      mask Type: Advanced_SmartMotorWrite
      mask Display:
      | color('white');
      | plot([100,100,100,100]*1,[100,100,100,100]*1);
      | plot([100,100,100,100]*0,[100,100,100,100]*0);
      | color('black');
      | image(fullfile(codertarget.vexv5.internal.getSpPkgRootDir, 'resources', 'vex-v5-motor2.png'),'center');
      | patch([0.8, 0.8, 1, 1], [0.82857, 1, 1, 0.82857], [1, 1, 1]);
      | color('blue');
      | text(99, 92, 'VEX V5 ', 'horizontalAlignment', 'right');
      | color('black');
      | text(62,12,'Port: 1','horizontalAlignment','center');
      | 
      | port_label('Input',1,'Voltage(mV)');
  wires:
  " Input"/1 -> Advanced_SmartMotorWrite/1

== system NeuromorphicDogGait_WalksBackwards/Smart Motor Controller4 ==
  " Input" : Inport
  Advanced_SmartMotorWrite : MATLABSystem  System=Advanced_SmartMotorWrite  motorPort=11  scaleFactor=36:1  MotorBrakeMode=Coast  OperationMode=Advanced Control
      mask Type: Advanced_SmartMotorWrite
      mask Display:
      | color('white');
      | plot([100,100,100,100]*1,[100,100,100,100]*1);
      | plot([100,100,100,100]*0,[100,100,100,100]*0);
      | color('black');
      | image(fullfile(codertarget.vexv5.internal.getSpPkgRootDir, 'resources', 'vex-v5-motor2.png'),'center');
      | patch([0.8, 0.8, 1, 1], [0.82857, 1, 1, 0.82857], [1, 1, 1]);
      | color('blue');
      | text(99, 92, 'VEX V5 ', 'horizontalAlignment', 'right');
      | color('black');
      | text(62,12,'Port: 11','horizontalAlignment','center');
      | 
      | port_label('Input',1,'Voltage(mV)');
  wires:
  " Input"/1 -> Advanced_SmartMotorWrite/1

== system NeuromorphicDogGait_WalksBackwards/Smart Motor Controller5 ==
  " Input" : Inport
  Advanced_SmartMotorWrite : MATLABSystem  System=Advanced_SmartMotorWrite  motorPort=2  scaleFactor=36:1  MotorBrakeMode=Coast  OperationMode=Advanced Control
      mask Type: Advanced_SmartMotorWrite
      mask Display:
      | color('white');
      | plot([100,100,100,100]*1,[100,100,100,100]*1);
      | plot([100,100,100,100]*0,[100,100,100,100]*0);
      | color('black');
      | image(fullfile(codertarget.vexv5.internal.getSpPkgRootDir, 'resources', 'vex-v5-motor2.png'),'center');
      | patch([0.8, 0.8, 1, 1], [0.82857, 1, 1, 0.82857], [1, 1, 1]);
      | color('blue');
      | text(99, 92, 'VEX V5 ', 'horizontalAlignment', 'right');
      | color('black');
      | text(62,12,'Port: 2','horizontalAlignment','center');
      | 
      | port_label('Input',1,'Voltage(mV)');
  wires:
  " Input"/1 -> Advanced_SmartMotorWrite/1

== system NeuromorphicDogGait_WalksBackwards/Smart Motor Controller6 ==
  " Input" : Inport
  Advanced_SmartMotorWrite : MATLABSystem  System=Advanced_SmartMotorWrite  motorPort=12  scaleFactor=36:1  MotorBrakeMode=Coast  OperationMode=Advanced Control
      mask Type: Advanced_SmartMotorWrite
      mask Display:
      | color('white');
      | plot([100,100,100,100]*1,[100,100,100,100]*1);
      | plot([100,100,100,100]*0,[100,100,100,100]*0);
      | color('black');
      | image(fullfile(codertarget.vexv5.internal.getSpPkgRootDir, 'resources', 'vex-v5-motor2.png'),'center');
      | patch([0.8, 0.8, 1, 1], [0.82857, 1, 1, 0.82857], [1, 1, 1]);
      | color('blue');
      | text(99, 92, 'VEX V5 ', 'horizontalAlignment', 'right');
      | color('black');
      | text(62,12,'Port: 12','horizontalAlignment','center');
      | 
      | port_label('Input',1,'Voltage(mV)');
  wires:
  " Input"/1 -> Advanced_SmartMotorWrite/1

== system NeuromorphicDogGait_WalksBackwards/Smart Motor Controller7 ==
  " Input" : Inport
  Advanced_SmartMotorWrite : MATLABSystem  System=Advanced_SmartMotorWrite  motorPort=10  scaleFactor=36:1  MotorBrakeMode=Coast  OperationMode=Advanced Control
      mask Type: Advanced_SmartMotorWrite
      mask Display:
      | color('white');
      | plot([100,100,100,100]*1,[100,100,100,100]*1);
      | plot([100,100,100,100]*0,[100,100,100,100]*0);
      | color('black');
      | image(fullfile(codertarget.vexv5.internal.getSpPkgRootDir, 'resources', 'vex-v5-motor2.png'),'center');
      | patch([0.8, 0.8, 1, 1], [0.82857, 1, 1, 0.82857], [1, 1, 1]);
      | color('blue');
      | text(99, 92, 'VEX V5 ', 'horizontalAlignment', 'right');
      | color('black');
      | text(62,12,'Port: 10','horizontalAlignment','center');
      | 
      | port_label('Input',1,'Voltage(mV)');
  wires:
  " Input"/1 -> Advanced_SmartMotorWrite/1

== system NeuromorphicDogGait_WalksBackwards/Smart Motor Controller8 ==
  " Input" : Inport
  Advanced_SmartMotorWrite : MATLABSystem  System=Advanced_SmartMotorWrite  motorPort=20  scaleFactor=36:1  MotorBrakeMode=Coast  OperationMode=Advanced Control
      mask Type: Advanced_SmartMotorWrite
      mask Display:
      | color('white');
      | plot([100,100,100,100]*1,[100,100,100,100]*1);
      | plot([100,100,100,100]*0,[100,100,100,100]*0);
      | color('black');
      | image(fullfile(codertarget.vexv5.internal.getSpPkgRootDir, 'resources', 'vex-v5-motor2.png'),'center');
      | patch([0.8, 0.8, 1, 1], [0.82857, 1, 1, 0.82857], [1, 1, 1]);
      | color('blue');
      | text(99, 92, 'VEX V5 ', 'horizontalAlignment', 'right');
      | color('black');
      | text(62,12,'Port: 20','horizontalAlignment','center');
      | 
      | port_label('Input',1,'Voltage(mV)');
  wires:
  " Input"/1 -> Advanced_SmartMotorWrite/1

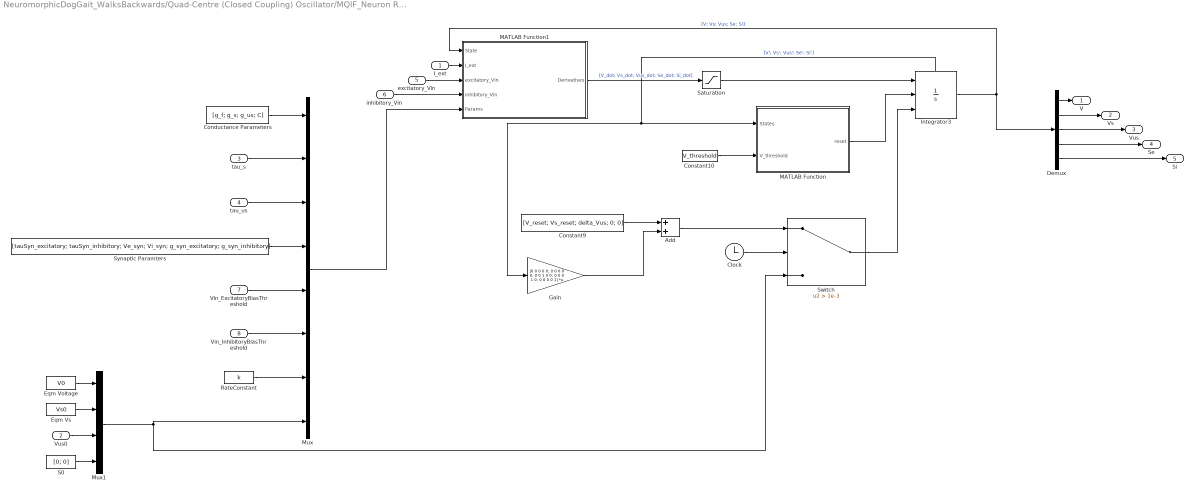
== system NeuromorphicDogGait_WalksBackwards/Quad-Centre (Closed Coupling) Oscillator/MQIF_Neuron Range of Motion Bounder A ==
  I_ext : Inport
  Vus0 : Inport  Port=2
  tau_s : Inport  Port=3
  tau_us : Inport  Port=4
  excitatory_Vin : Inport  Port=5
  inhibitory_Vin : Inport  Port=6
  Vin_ExcitatoryBiasThreshold : Inport  Port=7
  Vin_InhibitoryBiasThreshold : Inport  Port=8
  Add : Sum
  Clock : Clock
  Conductance Parameters : Constant  Value=[g_f; g_s; g_us; C]
  Constant10 : Constant  Value=V_threshold
  Constant9 : Constant  Value=[V_reset; Vs_reset; delta_Vus; 0; 0]
  Demux : Demux  Outputs=5
  Eqm Voltage : Constant  Value=V0
  Eqm Vs : Constant  Value=Vs0
  Gain : Gain  Gain=[0 0 0 0 0; 0 0 0 0 0; 0 0 1 0 0; 0 0 0 1 0; 0 0 0 0 1]  Multiplication=Matrix(K*u) (u vector)
  Integrator3 : Integrator  ExternalReset=rising  InitialConditionSource=external  InitialCondition=[V0 Vs0 Vus0]  ShowStatePort=on
  MATLAB Function : MATLAB Function  TreatAsAtomicUnit=on
  MATLAB Function1 : MATLAB Function  TreatAsAtomicUnit=on
  Mux : Mux  Inputs=8
  Mux1 : Mux
  RateConstant : Constant  Value=k
  S0 : Constant  Value=[0; 0]
  Saturation : Saturate  UpperLimit=1e4  LowerLimit=-1e4  LinearizeAsGain=off  ZeroCross=off
  Switch : Switch  Criteria=u2 > Threshold  Threshold=1e-3  SaturateOnIntegerOverflow=off  InputSameDT=off
  Synaptic Paramters : Constant  Value=[tauSyn_excitatory; tauSyn_inhibitory; Ve_syn; Vi_syn; g_syn_excitatory; g_syn_inhibitory]
  V : Outport
  Vs : Outport  Port=2
  Vus : Outport  Port=3
  Se : Outport  Port=4
  Si : Outport  Port=5
  wires:
  I_ext/1 -> MATLAB Function1/2(I_ext)
  Eqm Voltage/1 -> Mux1/1
  Vus0/1 -> Mux1/3
  Conductance Parameters/1 -> Mux/1
  tau_s/1 -> Mux/2
  tau_us/1 -> Mux/3
  Synaptic Paramters/1 -> Mux/4
  Mux/1 -> MATLAB Function1/5(Params)
  Constant10/1 -> MATLAB Function/2(V_threshold)
  Integrator3/1 -> MATLAB Function1/1(State), Demux/1  "[V; Vs; Vus; Se; Si]"
  Demux/1 -> V/1
  Demux/2 -> Vs/1
  Demux/3 -> Vus/1
  MATLAB Function/1(reset) -> Integrator3/2
  Clock/1 -> Switch/2
  Constant9/1 -> Add/1
  Switch/1 -> Integrator3/3
  Gain/1 -> Add/2
  MATLAB Function1/1(Derivatives) -> Saturation/1  "[V_dot; Vs_dot; Vus_dot; Se_dot; Si_dot]"
  Add/1 -> Switch/1
  Eqm Vs/1 -> Mux1/2
  inhibitory_Vin/1 -> MATLAB Function1/4(inhibitory_Vin)
  S0/1 -> Mux1/4
  Integrator3/State -> Gain/1, MATLAB Function/1(States)  "[V'; Vs'; Vus'; Se'; Si']"
  Demux/4 -> Se/1
  Vin_ExcitatoryBiasThreshold/1 -> Mux/5
  Saturation/1 -> Integrator3/1
  excitatory_Vin/1 -> MATLAB Function1/3(excitatory_Vin)
  Demux/5 -> Si/1
  RateConstant/1 -> Mux/7
  Mux1/1 -> Mux/8, Switch/3
  Vin_InhibitoryBiasThreshold/1 -> Mux/6

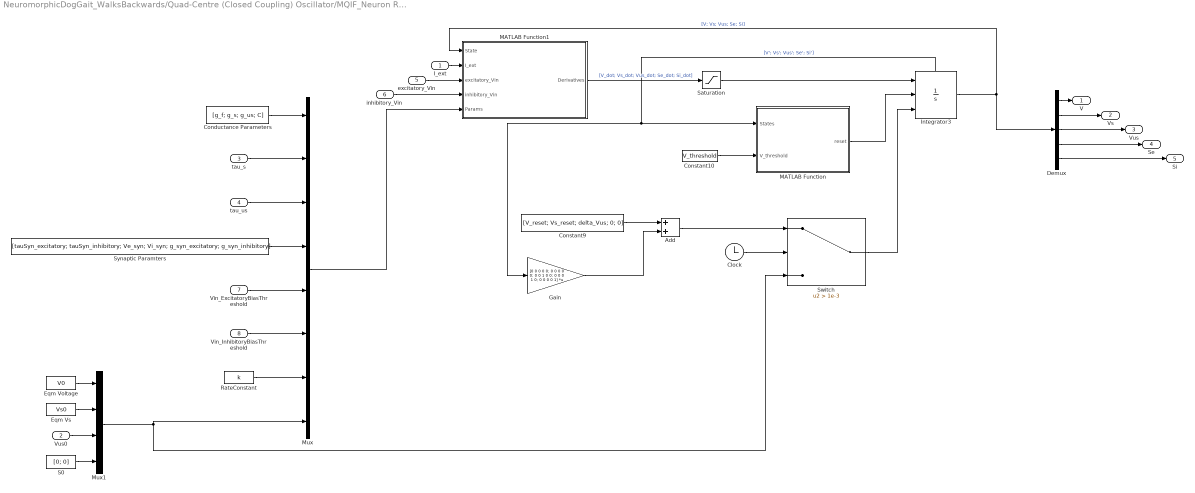
== system NeuromorphicDogGait_WalksBackwards/Quad-Centre (Closed Coupling) Oscillator/MQIF_Neuron Range of Motion Bounder B ==
  I_ext : Inport
  Vus0 : Inport  Port=2
  tau_s : Inport  Port=3
  tau_us : Inport  Port=4
  excitatory_Vin : Inport  Port=5
  inhibitory_Vin : Inport  Port=6
  Vin_ExcitatoryBiasThreshold : Inport  Port=7
  Vin_InhibitoryBiasThreshold : Inport  Port=8
  Add : Sum
  Clock : Clock
  Conductance Parameters : Constant  Value=[g_f; g_s; g_us; C]
  Constant10 : Constant  Value=V_threshold
  Constant9 : Constant  Value=[V_reset; Vs_reset; delta_Vus; 0; 0]
  Demux : Demux  Outputs=5
  Eqm Voltage : Constant  Value=V0
  Eqm Vs : Constant  Value=Vs0
  Gain : Gain  Gain=[0 0 0 0 0; 0 0 0 0 0; 0 0 1 0 0; 0 0 0 1 0; 0 0 0 0 1]  Multiplication=Matrix(K*u) (u vector)
  Integrator3 : Integrator  ExternalReset=rising  InitialConditionSource=external  InitialCondition=[V0 Vs0 Vus0]  ShowStatePort=on
  MATLAB Function : MATLAB Function  TreatAsAtomicUnit=on
  MATLAB Function1 : MATLAB Function  TreatAsAtomicUnit=on
  Mux : Mux  Inputs=8
  Mux1 : Mux
  RateConstant : Constant  Value=k
  S0 : Constant  Value=[0; 0]
  Saturation : Saturate  UpperLimit=1e4  LowerLimit=-1e4  LinearizeAsGain=off  ZeroCross=off
  Switch : Switch  Criteria=u2 > Threshold  Threshold=1e-3  SaturateOnIntegerOverflow=off  InputSameDT=off
  Synaptic Paramters : Constant  Value=[tauSyn_excitatory; tauSyn_inhibitory; Ve_syn; Vi_syn; g_syn_excitatory; g_syn_inhibitory]
  V : Outport
  Vs : Outport  Port=2
  Vus : Outport  Port=3
  Se : Outport  Port=4
  Si : Outport  Port=5
  wires:
  I_ext/1 -> MATLAB Function1/2(I_ext)
  Eqm Voltage/1 -> Mux1/1
  Vus0/1 -> Mux1/3
  Conductance Parameters/1 -> Mux/1
  tau_s/1 -> Mux/2
  tau_us/1 -> Mux/3
  Synaptic Paramters/1 -> Mux/4
  Mux/1 -> MATLAB Function1/5(Params)
  Constant10/1 -> MATLAB Function/2(V_threshold)
  Integrator3/1 -> MATLAB Function1/1(State), Demux/1  "[V; Vs; Vus; Se; Si]"
  Demux/1 -> V/1
  Demux/2 -> Vs/1
  Demux/3 -> Vus/1
  MATLAB Function/1(reset) -> Integrator3/2
  Clock/1 -> Switch/2
  Constant9/1 -> Add/1
  Switch/1 -> Integrator3/3
  Gain/1 -> Add/2
  MATLAB Function1/1(Derivatives) -> Saturation/1  "[V_dot; Vs_dot; Vus_dot; Se_dot; Si_dot]"
  Add/1 -> Switch/1
  Eqm Vs/1 -> Mux1/2
  inhibitory_Vin/1 -> MATLAB Function1/4(inhibitory_Vin)
  S0/1 -> Mux1/4
  Integrator3/State -> Gain/1, MATLAB Function/1(States)  "[V'; Vs'; Vus'; Se'; Si']"
  Demux/4 -> Se/1
  Vin_ExcitatoryBiasThreshold/1 -> Mux/5
  Saturation/1 -> Integrator3/1
  excitatory_Vin/1 -> MATLAB Function1/3(excitatory_Vin)
  Demux/5 -> Si/1
  RateConstant/1 -> Mux/7
  Mux1/1 -> Mux/8, Switch/3
  Vin_InhibitoryBiasThreshold/1 -> Mux/6

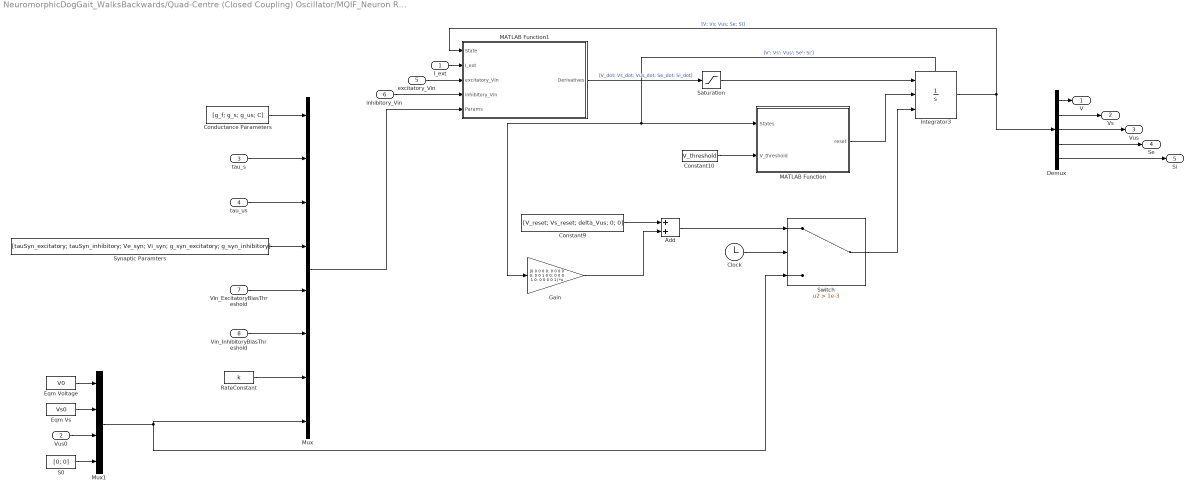
== system NeuromorphicDogGait_WalksBackwards/Quad-Centre (Closed Coupling) Oscillator/MQIF_Neuron Range of Motion Bounder C ==
  I_ext : Inport
  Vus0 : Inport  Port=2
  tau_s : Inport  Port=3
  tau_us : Inport  Port=4
  excitatory_Vin : Inport  Port=5
  inhibitory_Vin : Inport  Port=6
  Vin_ExcitatoryBiasThreshold : Inport  Port=7
  Vin_InhibitoryBiasThreshold : Inport  Port=8
  Add : Sum
  Clock : Clock
  Conductance Parameters : Constant  Value=[g_f; g_s; g_us; C]
  Constant10 : Constant  Value=V_threshold
  Constant9 : Constant  Value=[V_reset; Vs_reset; delta_Vus; 0; 0]
  Demux : Demux  Outputs=5
  Eqm Voltage : Constant  Value=V0
  Eqm Vs : Constant  Value=Vs0
  Gain : Gain  Gain=[0 0 0 0 0; 0 0 0 0 0; 0 0 1 0 0; 0 0 0 1 0; 0 0 0 0 1]  Multiplication=Matrix(K*u) (u vector)
  Integrator3 : Integrator  ExternalReset=rising  InitialConditionSource=external  InitialCondition=[V0 Vs0 Vus0]  ShowStatePort=on
  MATLAB Function : MATLAB Function  TreatAsAtomicUnit=on
  MATLAB Function1 : MATLAB Function  TreatAsAtomicUnit=on
  Mux : Mux  Inputs=8
  Mux1 : Mux
  RateConstant : Constant  Value=k
  S0 : Constant  Value=[0; 0]
  Saturation : Saturate  UpperLimit=1e4  LowerLimit=-1e4  LinearizeAsGain=off  ZeroCross=off
  Switch : Switch  Criteria=u2 > Threshold  Threshold=1e-3  SaturateOnIntegerOverflow=off  InputSameDT=off
  Synaptic Paramters : Constant  Value=[tauSyn_excitatory; tauSyn_inhibitory; Ve_syn; Vi_syn; g_syn_excitatory; g_syn_inhibitory]
  V : Outport
  Vs : Outport  Port=2
  Vus : Outport  Port=3
  Se : Outport  Port=4
  Si : Outport  Port=5
  wires:
  I_ext/1 -> MATLAB Function1/2(I_ext)
  Eqm Voltage/1 -> Mux1/1
  Vus0/1 -> Mux1/3
  Conductance Parameters/1 -> Mux/1
  tau_s/1 -> Mux/2
  tau_us/1 -> Mux/3
  Synaptic Paramters/1 -> Mux/4
  Mux/1 -> MATLAB Function1/5(Params)
  Constant10/1 -> MATLAB Function/2(V_threshold)
  Integrator3/1 -> MATLAB Function1/1(State), Demux/1  "[V; Vs; Vus; Se; Si]"
  Demux/1 -> V/1
  Demux/2 -> Vs/1
  Demux/3 -> Vus/1
  MATLAB Function/1(reset) -> Integrator3/2
  Clock/1 -> Switch/2
  Constant9/1 -> Add/1
  Switch/1 -> Integrator3/3
  Gain/1 -> Add/2
  MATLAB Function1/1(Derivatives) -> Saturation/1  "[V_dot; Vs_dot; Vus_dot; Se_dot; Si_dot]"
  Add/1 -> Switch/1
  Eqm Vs/1 -> Mux1/2
  inhibitory_Vin/1 -> MATLAB Function1/4(inhibitory_Vin)
  S0/1 -> Mux1/4
  Integrator3/State -> Gain/1, MATLAB Function/1(States)  "[V'; Vs'; Vus'; Se'; Si']"
  Demux/4 -> Se/1
  Vin_ExcitatoryBiasThreshold/1 -> Mux/5
  Saturation/1 -> Integrator3/1
  excitatory_Vin/1 -> MATLAB Function1/3(excitatory_Vin)
  Demux/5 -> Si/1
  RateConstant/1 -> Mux/7
  Mux1/1 -> Mux/8, Switch/3
  Vin_InhibitoryBiasThreshold/1 -> Mux/6

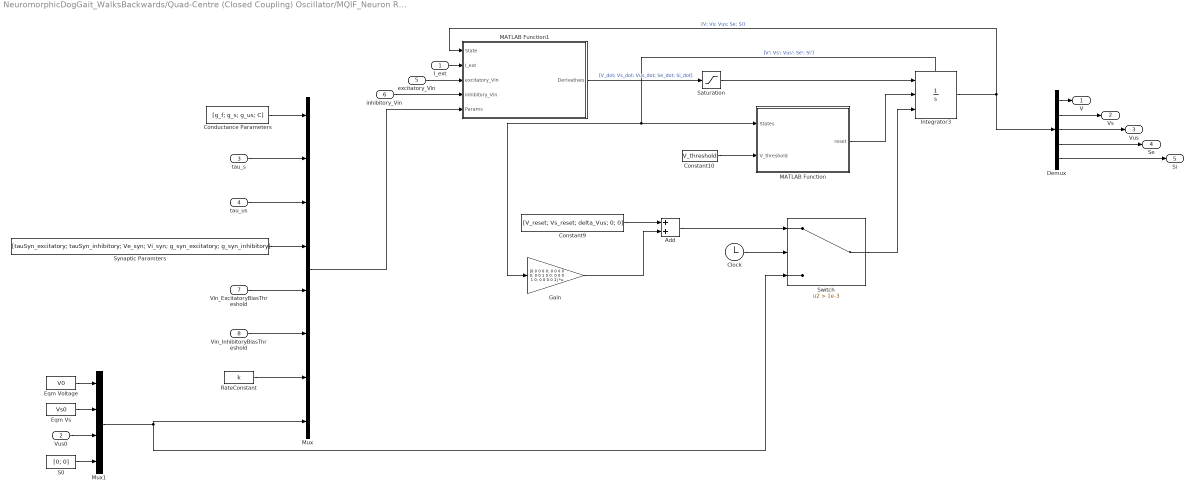
== system NeuromorphicDogGait_WalksBackwards/Quad-Centre (Closed Coupling) Oscillator/MQIF_Neuron Range of Motion Bounder D ==
  I_ext : Inport
  Vus0 : Inport  Port=2
  tau_s : Inport  Port=3
  tau_us : Inport  Port=4
  excitatory_Vin : Inport  Port=5
  inhibitory_Vin : Inport  Port=6
  Vin_ExcitatoryBiasThreshold : Inport  Port=7
  Vin_InhibitoryBiasThreshold : Inport  Port=8
  Add : Sum
  Clock : Clock
  Conductance Parameters : Constant  Value=[g_f; g_s; g_us; C]
  Constant10 : Constant  Value=V_threshold
  Constant9 : Constant  Value=[V_reset; Vs_reset; delta_Vus; 0; 0]
  Demux : Demux  Outputs=5
  Eqm Voltage : Constant  Value=V0
  Eqm Vs : Constant  Value=Vs0
  Gain : Gain  Gain=[0 0 0 0 0; 0 0 0 0 0; 0 0 1 0 0; 0 0 0 1 0; 0 0 0 0 1]  Multiplication=Matrix(K*u) (u vector)
  Integrator3 : Integrator  ExternalReset=rising  InitialConditionSource=external  InitialCondition=[V0 Vs0 Vus0]  ShowStatePort=on
  MATLAB Function : MATLAB Function  TreatAsAtomicUnit=on
  MATLAB Function1 : MATLAB Function  TreatAsAtomicUnit=on
  Mux : Mux  Inputs=8
  Mux1 : Mux
  RateConstant : Constant  Value=k
  S0 : Constant  Value=[0; 0]
  Saturation : Saturate  UpperLimit=1e4  LowerLimit=-1e4  LinearizeAsGain=off  ZeroCross=off
  Switch : Switch  Criteria=u2 > Threshold  Threshold=1e-3  SaturateOnIntegerOverflow=off  InputSameDT=off
  Synaptic Paramters : Constant  Value=[tauSyn_excitatory; tauSyn_inhibitory; Ve_syn; Vi_syn; g_syn_excitatory; g_syn_inhibitory]
  V : Outport
  Vs : Outport  Port=2
  Vus : Outport  Port=3
  Se : Outport  Port=4
  Si : Outport  Port=5
  wires:
  I_ext/1 -> MATLAB Function1/2(I_ext)
  Eqm Voltage/1 -> Mux1/1
  Vus0/1 -> Mux1/3
  Conductance Parameters/1 -> Mux/1
  tau_s/1 -> Mux/2
  tau_us/1 -> Mux/3
  Synaptic Paramters/1 -> Mux/4
  Mux/1 -> MATLAB Function1/5(Params)
  Constant10/1 -> MATLAB Function/2(V_threshold)
  Integrator3/1 -> MATLAB Function1/1(State), Demux/1  "[V; Vs; Vus; Se; Si]"
  Demux/1 -> V/1
  Demux/2 -> Vs/1
  Demux/3 -> Vus/1
  MATLAB Function/1(reset) -> Integrator3/2
  Clock/1 -> Switch/2
  Constant9/1 -> Add/1
  Switch/1 -> Integrator3/3
  Gain/1 -> Add/2
  MATLAB Function1/1(Derivatives) -> Saturation/1  "[V_dot; Vs_dot; Vus_dot; Se_dot; Si_dot]"
  Add/1 -> Switch/1
  Eqm Vs/1 -> Mux1/2
  inhibitory_Vin/1 -> MATLAB Function1/4(inhibitory_Vin)
  S0/1 -> Mux1/4
  Integrator3/State -> Gain/1, MATLAB Function/1(States)  "[V'; Vs'; Vus'; Se'; Si']"
  Demux/4 -> Se/1
  Vin_ExcitatoryBiasThreshold/1 -> Mux/5
  Saturation/1 -> Integrator3/1
  excitatory_Vin/1 -> MATLAB Function1/3(excitatory_Vin)
  Demux/5 -> Si/1
  RateConstant/1 -> Mux/7
  Mux1/1 -> Mux/8, Switch/3
  Vin_InhibitoryBiasThreshold/1 -> Mux/6
